simulink model "fixedPoint_model_q3_d"  (R2020b)
settings: Solver=FixedStepDiscrete  StartTime=0.0  StopTime=10  FixedStep=1/44100  RelTol=1e-3  EnableMultiTasking=on
settings Model: SILPILModeSetting=veronly  ExtModeTrigDuration=2  Creator=Faridodin  LastModifiedBy=Faridodin
settings OptimizationCC: EnhancedBackFolding=on  PassReuseOutputArgsAs=Individual arguments  ZeroExternalMemoryAtStartup=off  ZeroInternalMemoryAtStartup=off  MaxStackSize=64  OptimizeBlockOrder=speed  DifferentSizesBufferReuse=on  OptimizationCustomize=off  EfficientTunableParamExpr=on
settings DebuggingCC: SignalRangeChecking=warning  ParameterTunabilityLossMsg=error
settings HardwareCC: ProdBitPerInt=16  ProdBitPerPointer=16  ProdBitPerSizeT=16  ProdBitPerPtrDiffT=16  ProdLargestAtomicFloat=None  ProdWordSize=8  ProdHWDeviceType=Atmel->AVR
settings SFSimCC: MATLABDynamicMemAlloc=off
settings RTWCC: Description=Embedded Coder  SystemTargetFile=ert.tlc  HardwareBoard=Arduino Mega 2560  TemplateMakefile=ert_default_tmf  Toolchain=Arduino AVR  BuildConfiguration=Faster Runs
settings CodeAppCC: ForceParamTrailComments=on  IgnoreCustomStorageClasses=off  OperatorAnnotations=on  SimulinkDataObjDesc=on  SFDataObjDesc=on  InsertBlockDesc=on
settings ERTTargetCC: SupportContinuousTime=on  SupportVariableSizeSignals=on  ExtModeStaticAllocSize=2048

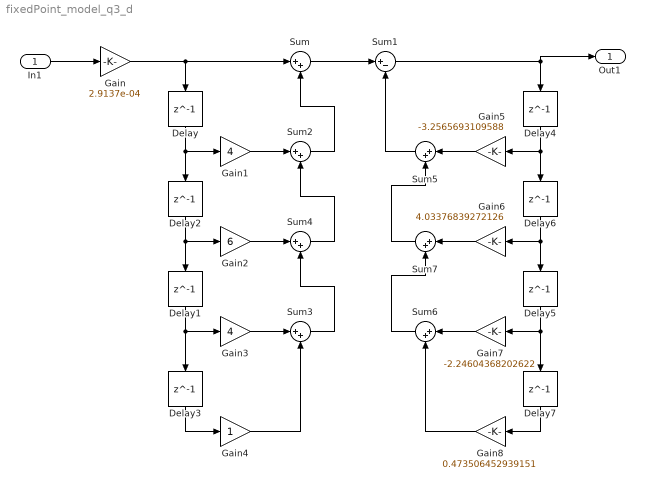
== system fixedPoint_model_q3_d ==
  In1 : Inport  OutDataTypeStr=fixdt(1,16,4)
  Delay{,1..7} (8 alike) : Delay  DelayLength=1  InitialCondition=0
  Gain : Gain  Gain=2.9137e-04  OutDataTypeStr=fixdt(1,16,4)
  Gain1 : Gain  Gain=4  OutDataTypeStr=fixdt(1,16,4)
  Gain2 : Gain  Gain=6  OutDataTypeStr=fixdt(1,16,4)
  Gain3 : Gain  Gain=4  OutDataTypeStr=fixdt(1,16,4)
  Gain4 : Gain  OutDataTypeStr=fixdt(1,16,4)
  Gain5 : Gain  Gain=-3.2565693109588  OutDataTypeStr=fixdt(1,16,4)
  Gain6 : Gain  Gain=4.03376839272126  OutDataTypeStr=fixdt(1,16,4)
  Gain7 : Gain  Gain=-2.24604368202622  OutDataTypeStr=fixdt(1,16,4)
  Gain8 : Gain  Gain=0.473506452939151  OutDataTypeStr=fixdt(1,16,4)
  Sum{,2..7} (7 alike) : Sum  Inputs=|++  OutDataTypeStr=fixdt(1,16,4)
  Sum1 : Sum  Inputs=|+-  OutDataTypeStr=fixdt(1,16,4)
  Out1 : Outport
  wires:
  Gain/1 -> Sum/1, Delay/1
  Delay3/1 -> Gain4/1
  Delay7/1 -> Gain8/1
  Gain2/1 -> Sum4/1
  Sum/1 -> Sum1/1
  Delay6/1 -> Delay5/1, Gain6/1
  Sum2/1 -> Sum/2
  Sum7/1 -> Sum5/2
  Sum3/1 -> Sum4/2
  Sum4/1 -> Sum2/2
  Sum1/1 -> Out1/1, Delay4/1
  Sum6/1 -> Sum7/2
  Delay4/1 -> Delay6/1, Gain5/1
  Delay1/1 -> Delay3/1, Gain3/1
  Gain5/1 -> Sum5/1
  Delay/1 -> Delay2/1, Gain1/1
  Gain1/1 -> Sum2/1
  Delay2/1 -> Delay1/1, Gain2/1
  Gain4/1 -> Sum3/2
  Sum5/1 -> Sum1/2
  Gain7/1 -> Sum6/1
  Gain6/1 -> Sum7/1
  Gain8/1 -> Sum6/2
  Gain3/1 -> Sum3/1
  Delay5/1 -> Delay7/1, Gain7/1
  In1/1 -> Gain/1
